simulink model "simulation"  (R2018a)
settings: Solver=VariableStepAuto  StartTime=0.0  StopTime=15  RelTol=1e-3
values from neighbouring files (symbols this model uses):
  A = [A1 zeros(2,2);zeros(2,2) A2]    [project.m]
  B = [B1 zeros(2,1);zeros(2,1) B2]    [project.m]
  C = [C1 C2]    [project.m]
  L = place(A',C', polesobserver)'    [project.m]
undefined symbols (not defined in the file or in its folder): KK
settings Model: Creator=Migue  LastModifiedBy=Migue

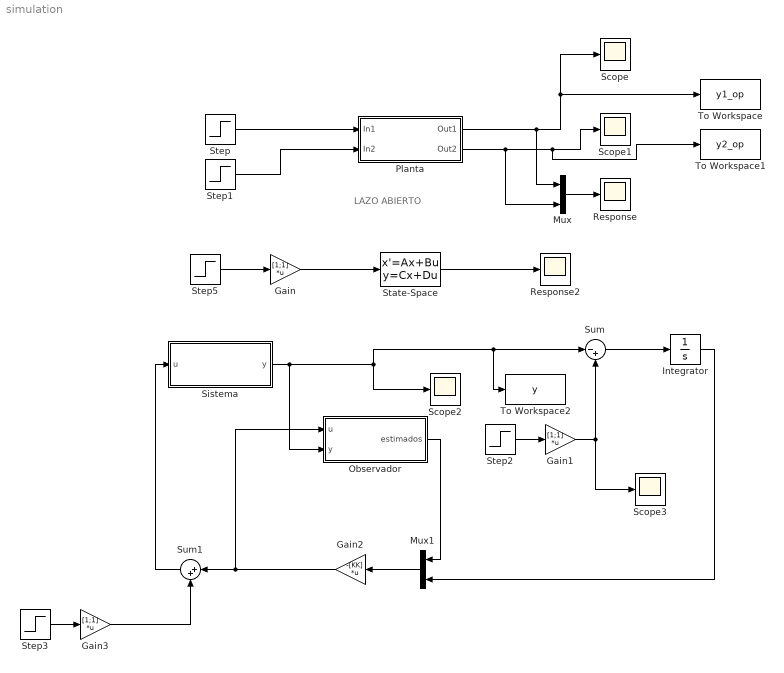
== system simulation ==
  note: LAZO ABIERTO
  Gain : Gain  Gain=[1;1]  Multiplication=Matrix(K*u)
  Gain1 : Gain  Gain=[1;1]  Multiplication=Matrix(K*u)
  Gain2 : Gain  Gain=-[KK]  Multiplication=Matrix(K*u)
  Gain3 : Gain  Gain=[1;1]  Multiplication=Matrix(K*u)
  Integrator : Integrator
  Mux : Mux  Inputs=2
  Mux1 : Mux  Inputs=2
  Observador : Subsystem
  Planta : Subsystem
  Response : Scope
  Response2 : Scope
  Scope{,1..3} (4 alike) : Scope
  Sistema : Subsystem
  State-Space : StateSpace  A=A  B=B  C=C  D=[0 0;0 0]  InitialCondition=0
  Step{,1..2,5} (4 alike) : Step  SampleTime=0
  Step3 : Step  Time=10  SampleTime=0
  Sum : Sum  Inputs=|-+
  Sum1 : Sum  Inputs=|++
  To Workspace : ToWorkspace  VariableName=y1_op  SaveFormat=Timeseries  SampleTime=-1
  To Workspace1 : ToWorkspace  VariableName=y2_op  SaveFormat=Timeseries  SampleTime=-1
  To Workspace2 : ToWorkspace  VariableName=y  SampleTime=-1
      settings: Save2DSignal=2-D array (concatenate along first dimension)
  wires:
  Step1/1 -> Planta/2(In2)
  Step/1 -> Planta/1(In1)
  Planta/2(Out2) -> Mux/2, To Workspace1/1, Scope1/1
  Planta/1(Out1) -> Mux/1, To Workspace/1, Scope/1
  Mux/1 -> Response/1
  State-Space/1 -> Response2/1
  Step5/1 -> Gain/1
  Gain/1 -> State-Space/1
  Gain1/1 -> Scope3/1, Sum/2
  Step2/1 -> Gain1/1
  Sum/1 -> Integrator/1
  Mux1/1 -> Gain2/1
  Observador/1(estimados) -> Mux1/1
  Integrator/1 -> Mux1/2
  Gain2/1 -> Sum1/1, Observador/1(u)
  Sistema/1(y) -> Scope2/1, To Workspace2/1, Sum/1, Observador/2(y)
  Sum1/1 -> Sistema/1(u)
  Step3/1 -> Gain3/1
  Gain3/1 -> Sum1/2

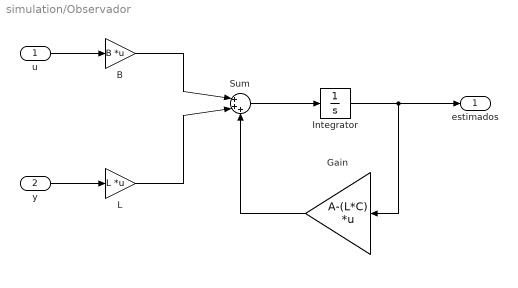
== system simulation/Observador ==
  u : Inport
  y : Inport  Port=2
  B : Gain  Gain=B  Multiplication=Matrix(K*u)
  Gain : Gain  Gain=A-(L*C)  Multiplication=Matrix(K*u)
  Integrator : Integrator
  L : Gain  Gain=L  Multiplication=Matrix(K*u)
  Sum : Sum  Inputs=|+++
  estimados : Outport
  wires:
  u/1 -> B/1
  y/1 -> L/1
  B/1 -> Sum/1
  L/1 -> Sum/2
  Gain/1 -> Sum/3
  Sum/1 -> Integrator/1
  Integrator/1 -> Gain/1, estimados/1

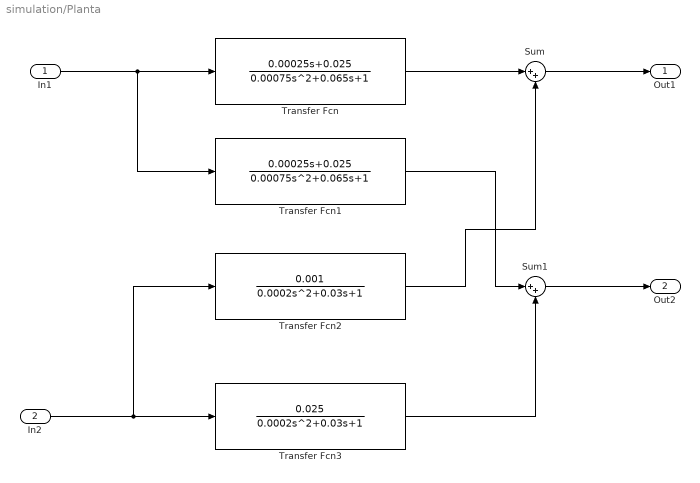
== system simulation/Planta ==
  In1 : Inport
  In2 : Inport  Port=2
  Sum : Sum  Inputs=|++
  Sum1 : Sum  Inputs=|++
  Transfer Fcn : TransferFcn  Numerator=[0.00025 0.025]  Denominator=[0.00075 0.065 1]
  Transfer Fcn1 : TransferFcn  Numerator=[0.00025 0.025]  Denominator=[0.00075 0.065 1]
  Transfer Fcn2 : TransferFcn  Numerator=[0.001]  Denominator=[0.0002 0.03 1]
  Transfer Fcn3 : TransferFcn  Numerator=[0.025]  Denominator=[0.0002 0.03 1]
  Out1 : Outport
  Out2 : Outport  Port=2
  wires:
  In1/1 -> Transfer Fcn1/1, Transfer Fcn/1
  In2/1 -> Transfer Fcn3/1, Transfer Fcn2/1
  Transfer Fcn1/1 -> Sum1/1
  Transfer Fcn/1 -> Sum/1
  Transfer Fcn2/1 -> Sum/2
  Sum/1 -> Out1/1
  Transfer Fcn3/1 -> Sum1/2
  Sum1/1 -> Out2/1

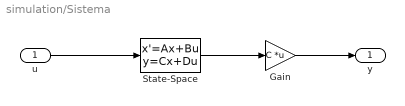
== system simulation/Sistema ==
  u : Inport
  Gain : Gain  Gain=C  Multiplication=Matrix(K*u)
  State-Space : StateSpace  A=A  B=B  C=eye(4)  D=zeros(4,2)  InitialCondition=0
  y : Outport
  wires:
  u/1 -> State-Space/1
  State-Space/1 -> Gain/1
  Gain/1 -> y/1
